simulink model "diagMA"  (R2024b)
settings: Solver=VariableStepAuto  StartTime=0.0  StopTime=simTime  RelTol=1e-3
values from neighbouring files (symbols this model uses):
  alpha = 1*pi/180    (= 0.0174532925199)    [setup.m]
  b = DH/roCp    (= -11.92)    [fsolve1.m]    (also in setup.m = 7)
  c = UA/roCp/V    (= 0.3)    [fsolve1.m]    (also in setup.m = 3)
  g = 9.8    [setup.m]
  m = 1200    [setup.m]
  Ts = 0.1    [simMA.m]
  uStep = 100*g    [simMA.m]
  v0 = 0    [simMA.m]
settings Model: Creator=marcelo  LastModifiedBy=marcelo
settings SolverCC: AlgebraicLoopSolver=TrustRegion
settings DataIOCC: ReturnWorkspaceOutputs=off
settings DebuggingCC: UnconnectedInputMsg=warning  UnconnectedOutputMsg=warning  UnconnectedLineMsg=warning  ArithmeticOperatorsInVariantConditions=warning
settings ModelReferenceCC: EnableRefExpFcnMdlSchedulingChecks=on
settings SFSimCC: CustomCodeUndefinedFunction=UseInterfaceOnly
settings RTWCC: GPUComputeCapability=3.5

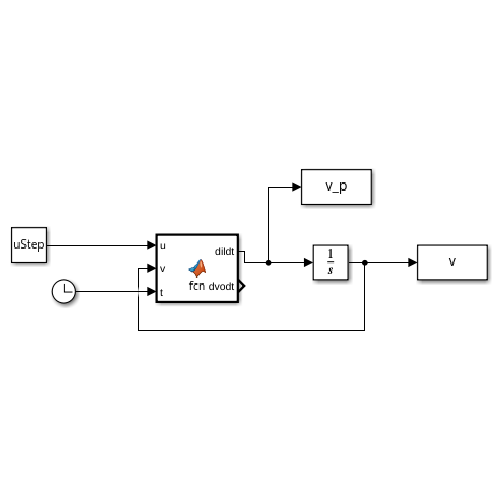
[thumbnail: Simulink's stored preview of the top-level diagram]
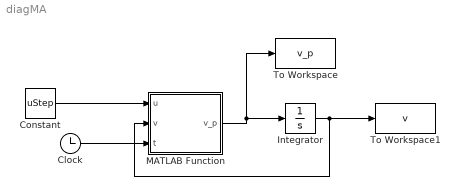
== system diagMA ==
  Clock : Clock
  Constant : Constant  Value=uStep  SampleTime=Ts
  Integrator : Integrator  InitialCondition=v0
  MATLAB Function : MATLAB Function  TreatAsAtomicUnit=on
  To Workspace : ToWorkspace  VariableName=v_p  SaveFormat=Timeseries  SampleTime=-1
  To Workspace1 : ToWorkspace  VariableName=v  SaveFormat=Timeseries  SampleTime=-1
  wires:
  Constant/1 -> MATLAB Function/1(u)
  MATLAB Function/1(v_p) -> To Workspace/1, Integrator/1
  Integrator/1 -> To Workspace1/1, MATLAB Function/2(v)
  Clock/1 -> MATLAB Function/3(t)

== matlab function diagMA/MATLAB Function ==
  settings: updateMethod=DISCRETE  sampleTime=Ts
  data: u input; v_p output; m parameter; c parameter; g parameter; v input; alpha parameter; b parameter; t input
function v_p  = fcn(u,m, c, g, v, alpha, b, t)

persistent t_OLD; % declaração da variável persistente (que retém o
                  %valor da última iteração

if isempty(t_OLD) % inicialização
    t_OLD = 0;
end

v_p = (1/m)*(u - b*v - c*(v^2) - m*g*sin(alpha));

Dt = t - t_OLD; %(exemplo) cálculo do período de amostragem desta função

t_OLD = t; % atualização da variável persistente

end
